simulink model "group7undergrad"  (R2024a)
settings: Solver=FixedStepAuto  StartTime=0.0  StopTime=100.0  RelTol=1e-3
libraries: robotlib x3
settings Model: Creator=katiegildersleeve  LastModifiedBy=katiegildersleeve
settings OptimizationCC: EnhancedBackFolding=on  PassReuseOutputArgsAs=Individual arguments  ZeroExternalMemoryAtStartup=off  ZeroInternalMemoryAtStartup=off  MaxStackSize=64  OptimizeBlockOrder=speed  DifferentSizesBufferReuse=on  OptimizationCustomize=off  EfficientTunableParamExpr=on
settings DebuggingCC: ParameterTunabilityLossMsg=error
settings HardwareCC: ProdBitPerPointer=32  ProdBitPerSizeT=32  ProdBitPerPtrDiffT=32  ProdLargestAtomicFloat=None  ProdIntDivRoundTo=Undefined  ProdEndianess=Unspecified  ProdWordSize=32  ProdHWDeviceType=Generic->Unspecified (assume 32-bit Generic)  UseEmbeddedCoderFeatures=off
settings SFSimCC: MATLABDynamicMemAlloc=off
settings RTWCC: Description=Embedded Coder  SystemTargetFile=ert.tlc  HardwareBoard=Robot Operating System (ROS)  TLCOptions="-aInlineSetEventsForThisBaseRateFcn=TLC_FALSE -aSuppressMultiTaskScheduler=TLC_FALSE  -aRateBasedStepFcn=0"  TemplateMakefile=ert_default_tmf  Toolchain=Catkin  TargetLang=C++
settings CodeAppCC: ForceParamTrailComments=on  IgnoreCustomStorageClasses=off  OperatorAnnotations=on  SimulinkDataObjDesc=on  SFDataObjDesc=on  InsertBlockDesc=on
settings ERTTargetCC: SupportNonInlinedSFcns=on

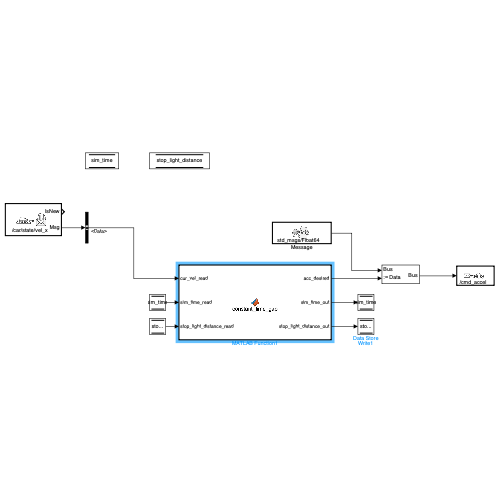
[thumbnail: Simulink's stored preview of the top-level diagram]
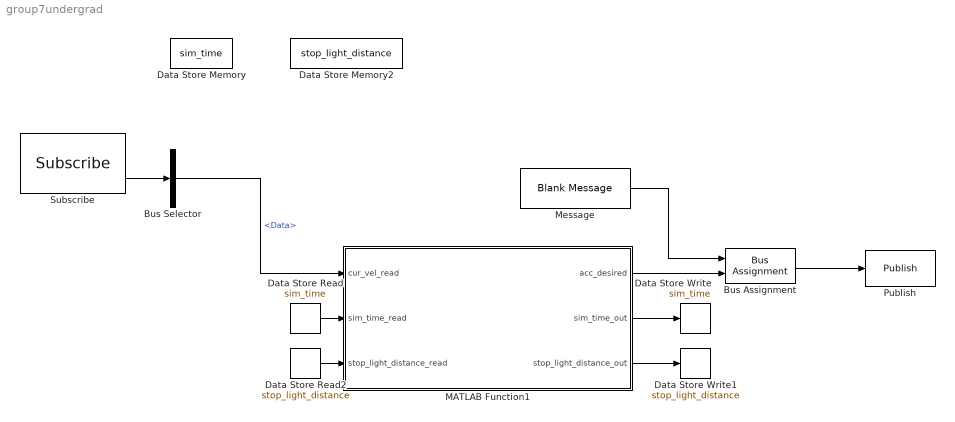
== system group7undergrad ==
  Bus Assignment : BusAssignment  AssignedSignals=Data
  Bus Selector : BusSelector  OutputSignals=Data
  Data Store Memory : DataStoreMemory  DataStoreName=sim_time  WriteAfterWriteMsg=warning  ShowAdditionalParam=off  OutDataTypeStr=double  Dimensions=1
  Data Store Memory2 : DataStoreMemory  DataStoreName=stop_light_distance  WriteAfterWriteMsg=warning  InitialValue=500  ShowAdditionalParam=off  OutDataTypeStr=double
  Data Store Read : DataStoreRead  DataStoreName=sim_time  IndexOptions=Index vector (dialog)  Indices=1  OutputSizes=1
  Data Store Read2 : DataStoreRead  DataStoreName=stop_light_distance  DataStoreElements=stop_light_distance  IndexOptions=Index vector (dialog)  Indices=1  OutputSizes=1
  Data Store Write : DataStoreWrite  DataStoreName=sim_time  IndexOptions=Index vector (dialog)  Indices=1  OutputSizes=1
  Data Store Write1 : DataStoreWrite  DataStoreName=stop_light_distance  DataStoreElements=stop_light_distance  IndexOptions=Index vector (dialog)  Indices=1  OutputSizes=1
  MATLAB Function1 : MATLAB Function  TreatAsAtomicUnit=on
  Message : robotlib/Blank Message  messageClass=Message  entityType=std_msgs/Float64  messageType=std_msgs/Float64  SampleTime=inf  legacyBusStruct=off
  Publish : robotlib/Publish  topicSource=Specify your own  topic=/cmd_accel  messageType=std_msgs/Float64  legacyBusStruct=off  messageQueueLength=1
  Subscribe : robotlib/Subscribe  topicSource=Specify your own  topic=/car/state/vel_x  messageType=std_msgs/Float64  SampleTime=-1  legacyBusStruct=off  messageQueueLength=1
  wires:
  Message/1 -> Bus Assignment/1
  Bus Assignment/1 -> Publish/1
  MATLAB Function1/1(acc_desired) -> Bus Assignment/2
  Data Store Read/1 -> MATLAB Function1/2(sim_time_read)
  MATLAB Function1/2(sim_time_out) -> Data Store Write/1
  Data Store Read2/1 -> MATLAB Function1/3(stop_light_distance_read)
  MATLAB Function1/3(stop_light_distance_out) -> Data Store Write1/1
  Subscribe/2 -> Bus Selector/1
  Bus Selector/1 -> MATLAB Function1/1(cur_vel_read)  "<Data>"

== matlab function group7undergrad/MATLAB Function1 ==
  data: cur_vel_read input; sim_time_read input; acc_desired output; sim_time_out output; stop_light_distance_read input; stop_light_distance_out output
function [acc_desired, sim_time_out, stop_light_distance_out] = constant_time_gap(cur_vel_read, sim_time_read, stop_light_distance_read)
    % Read the current simulation time and stop light distance from input
    time_step = 1;
    sim_time = sim_time_read;
    stop_light_distance = stop_light_distance_read;
    vel_ego = cur_vel_read;

    % Traffic Light Timing
    time_to_green = 40 - sim_time;  % Time until the light turns green

    % Control Parameters
    alpha = 0.25;         % Control gain

    % Update the distance to the stoplight based on velocity
    stop_light_distance = stop_light_distance - (vel_ego * time_step);

    % Check for critical distance to the lead vehicle (space_gap) or stoplight
    critical_distance_to_stoplight = 100;    % Distance to start slowing down for the stoplight

    % If the lead vehicle is too close, prioritize avoiding a collision
    if stop_light_distance <= critical_distance_to_stoplight && time_to_green > 0
        % Approaching the stoplight while it's red
        % Calculate target velocity to arrive as the light turns green
        target_velocity = stop_light_distance / time_to_green;
        acc_desired = alpha * (target_velocity - vel_ego);
    else
        % Normal control behavior (no immediate lead vehicle or red light)
        acc_desired = alpha * (15 - vel_ego);
    end

    % Safety Check: Prevent negative or excessively high acceleration
    if stop_light_distance < 0
        acc_desired = alpha * (15 - vel_ego);  % Stop if too close to the stoplight
    end

    % Update the simulation time
    sim_time = sim_time + time_step;

    % Output the updated values
    sim_time_out = sim_time;
    stop_light_distance_out = stop_light_distance;
end
